simulink model "pendulum_control"  (R2025b)
settings: Solver=VariableStepAuto  StartTime=0.0  StopTime=4  RelTol=1e-3
undefined symbols (not defined in the file): b, K, Kd, Kp, Kt, L, R, setpoint
settings Model: Creator=REARDONNM24  LastModifiedBy=REARDONNM24

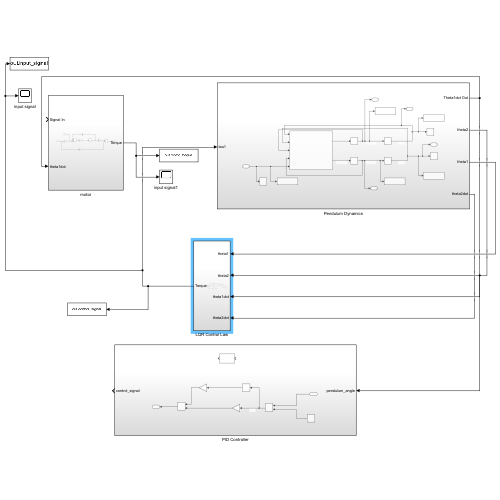
[thumbnail: Simulink's stored preview of the top-level diagram]
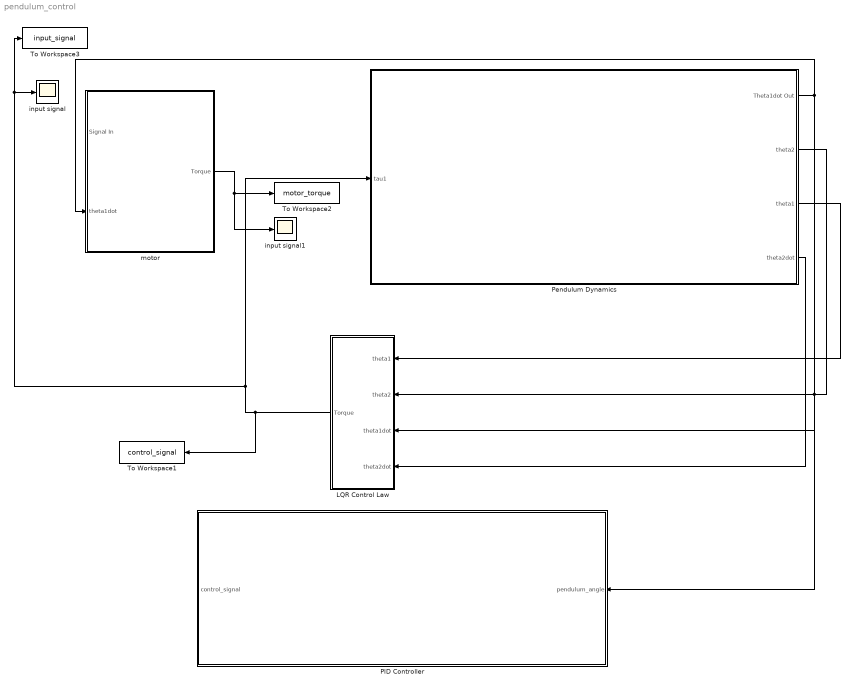
== system pendulum_control ==
  LQR Control Law : Subsystem
  PID Controller : Subsystem
      settings: PortSchema="{\"entries\":[{\"content\":{\"sides\":[{\"content\":{\"connectorIds\":[\"Out1\"]},\"type\":\"ConnectorPlacement.EquallySpacedRectSide\",\"uuid\":\"140972ef-afa4-4424-8e07-e9b39865205a\"},{\"content\":{\"connectorIds\":[\"In1\"],\"side\":\"RIGHT\"},\"type\":\"ConnectorPlacement.EquallySpacedRectSide\",\"uuid\":\"e18a6186-4364-4339-999d-66e09d6bd355\"},{\"content\":{\"side\":\"TOP\"},\"type\":\"ConnectorPlacement.EquallySpacedRectSide\",\"uuid\":\"cdbf3bcd-b810-497c-aa1d-b7994b8093ed\"}]},\"type\":\"ConnectorPlacement.EquallySpacedConnector\",\"uuid\":\"2c683edf-d322-406a-ba66-9fd9d67fa1ef\"}],\"packageUris\":[\"http://schema.mathworks.com/mf0/Connector/R2020b\"],\"version\":\"1.0\"}"
  Pendulum Dynamics : Subsystem
  To Workspace1 : ToWorkspace  VariableName=control_signal  SaveFormat=Timeseries  SampleTime=-1
  To Workspace2 : ToWorkspace  VariableName=motor_torque  SaveFormat=Timeseries  SampleTime=-1
  To Workspace3 : ToWorkspace  VariableName=input_signal  SaveFormat=Timeseries  SampleTime=-1
  input signal : Scope
      settings: ActiveDisplayYMinimum=174.41543511722466  ActiveDisplayYMaximum=4357.1108128089754  DataLoggingVariableName=ScopeData6
  input signal1 : Scope
      settings: ActiveDisplayYMinimum=-0.0033441907118329393  ActiveDisplayYMaximum=0.00610606731194419  DataLoggingVariableName=ScopeData7
  motor : Subsystem
  wires:
  Pendulum Dynamics/1(Theta1dot Out) -> motor/2(theta1dot), LQR Control Law/3(theta1dot)
  motor/1(Torque) -> input signal1/1, To Workspace2/1
  Pendulum Dynamics/2(theta2) -> LQR Control Law/2(theta2), PID Controller/1(pendulum_angle)
  Pendulum Dynamics/3(theta1) -> LQR Control Law/1(theta1)
  Pendulum Dynamics/4(theta2dot) -> LQR Control Law/4(theta2dot)
  LQR Control Law/1(Torque) -> To Workspace1/1, To Workspace3/1, input signal/1, Pendulum Dynamics/1(tau1)

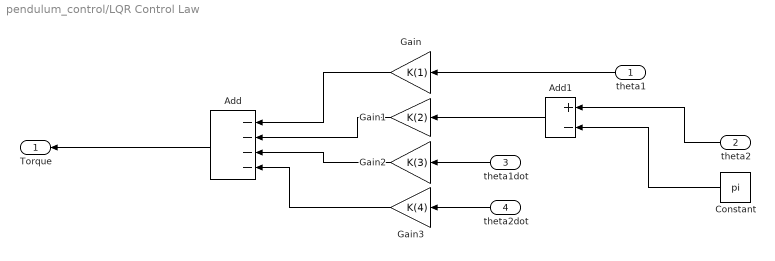
== system pendulum_control/LQR Control Law ==
  theta1 : Inport
  theta2 : Inport  Port=2
  theta1dot : Inport  Port=3
  theta2dot : Inport  Port=4
  Add : Sum  Inputs=----
  Add1 : Sum  Inputs=+-
  Constant : Constant  Value=pi
  Gain : Gain  Gain=K(1)
  Gain1 : Gain  Gain=K(2)
  Gain2 : Gain  Gain=K(3)
  Gain3 : Gain  Gain=K(4)
  Torque : Outport
  wires:
  Gain3/1 -> Add/4
  Gain/1 -> Add/1
  theta2dot/1 -> Gain3/1
  theta1dot/1 -> Gain2/1
  Gain1/1 -> Add/2
  Gain2/1 -> Add/3
  Add/1 -> Torque/1
  Constant/1 -> Add1/2
  theta2/1 -> Add1/1
  theta1/1 -> Gain/1
  Add1/1 -> Gain1/1

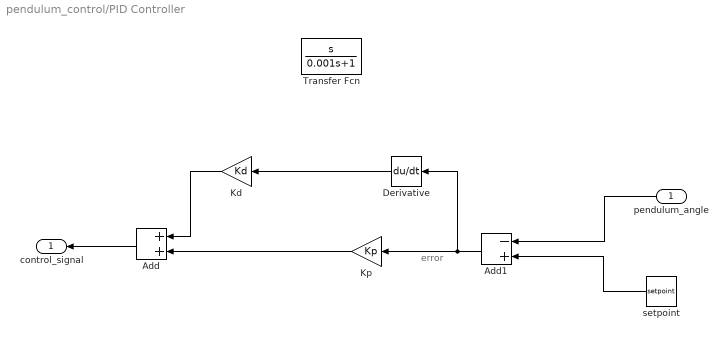
== system pendulum_control/PID Controller ==
  note: error
  pendulum_angle : Inport
  Add : Sum
  Add1 : Sum  Inputs=-+
  Derivative : Derivative
  Kd : Gain  Gain=Kd
  Kp : Gain  Gain=Kp
  Transfer Fcn : TransferFcn  Numerator=[1 0]  Denominator=[0.001 1]
  setpoint : Constant  Value=setpoint
  control_signal : Outport
  wires:
  Add1/1 -> Derivative/1, Kp/1
  setpoint/1 -> Add1/2
  pendulum_angle/1 -> Add1/1
  Kp/1 -> Add/2
  Kd/1 -> Add/1
  Add/1 -> control_signal/1
  Derivative/1 -> Kd/1

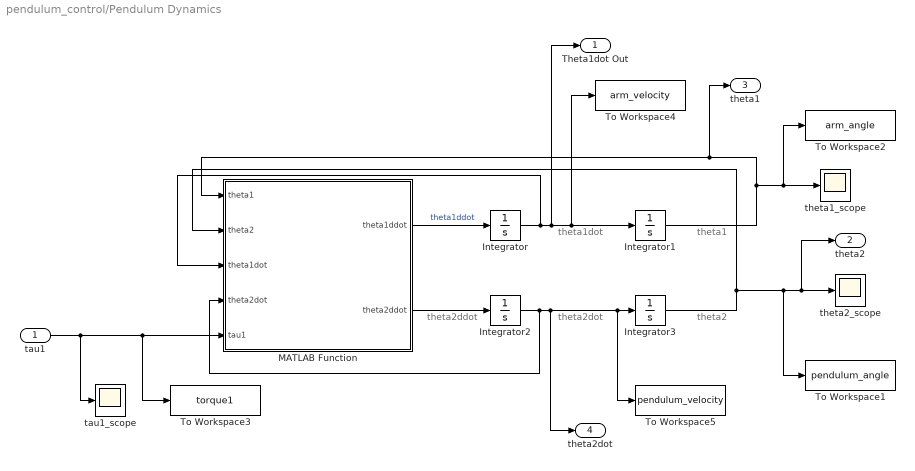
== system pendulum_control/Pendulum Dynamics ==
  note: theta1
  note: theta2
  note: theta2dot
  note: theta2ddot
  note: theta1dot
  tau1 : Inport
  Integrator : Integrator
  Integrator1 : Integrator
  Integrator2 : Integrator
  Integrator3 : Integrator  InitialCondition=2.96
  MATLAB Function : MATLAB Function  TreatAsAtomicUnit=on
  To Workspace1 : ToWorkspace  VariableName=pendulum_angle  SaveFormat=Timeseries  SampleTime=-1
  To Workspace2 : ToWorkspace  VariableName=arm_angle  SaveFormat=Timeseries  SampleTime=-1
  To Workspace3 : ToWorkspace  VariableName=torque1  SaveFormat=Timeseries  SampleTime=-1
  To Workspace4 : ToWorkspace  VariableName=arm_velocity  SaveFormat=Timeseries  SampleTime=-1
  To Workspace5 : ToWorkspace  VariableName=pendulum_velocity  SaveFormat=Timeseries  SampleTime=-1
  tau1_scope : Scope
      settings: ActiveDisplayYMinimum=-0.018770395001535239  ActiveDisplayYMaximum=0.012159767110327464  DataLoggingVariableName=ScopeData4
  theta1_scope : Scope
      settings: ActiveDisplayYMinimum=-0.0042282998397400089  ActiveDisplayYMaximum=0.03805469855766009  DataLoggingVariableName=ScopeData2
  theta2_scope : Scope
      settings: ActiveDisplayYMinimum=-1.85410777692418  ActiveDisplayYMaximum=-0.63109346273532874  DataLoggingVariableName=ScopeData3
  Theta1dot Out : Outport
  theta2 : Outport  Port=2
  theta1 : Outport  Port=3
  theta2dot : Outport  Port=4
  wires:
  MATLAB Function/1(theta1ddot) -> Integrator/1  "theta1ddot"
  Integrator/1 -> MATLAB Function/3(theta1dot), Theta1dot Out/1, Integrator1/1, To Workspace4/1
  Integrator2/1 -> MATLAB Function/4(theta2dot), theta2dot/1, To Workspace5/1, Integrator3/1
  MATLAB Function/2(theta2ddot) -> Integrator2/1
  Integrator3/1 -> To Workspace1/1, theta2/1, theta2_scope/1, MATLAB Function/2(theta2)
  Integrator1/1 -> To Workspace2/1, theta1_scope/1, theta1/1, MATLAB Function/1(theta1)
  tau1/1 -> tau1_scope/1, To Workspace3/1, MATLAB Function/5(tau1)

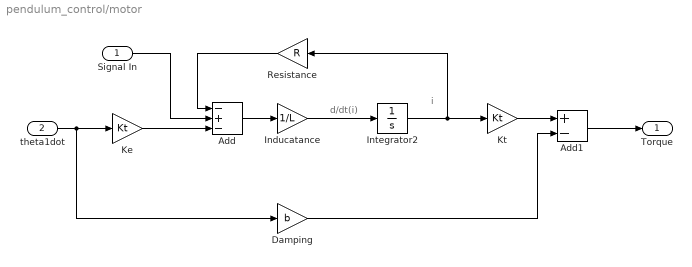
== system pendulum_control/motor ==
  note: i
  note: d/dt(i)
  Signal In : Inport
  theta1dot : Inport  Port=2
  Add : Sum  Inputs=-+-
  Add1 : Sum  Inputs=+-
  Damping : Gain  Gain=b
  Inducatance : Gain  Gain=1/L
  Integrator2 : Integrator
  Ke : Gain  Gain=Kt
  Kt : Gain  Gain=Kt
  Resistance : Gain  Gain=R
  Torque : Outport
  wires:
  Signal In/1 -> Add/2
  Resistance/1 -> Add/1
  Integrator2/1 -> Kt/1, Resistance/1
  Inducatance/1 -> Integrator2/1
  Add/1 -> Inducatance/1
  Ke/1 -> Add/3
  theta1dot/1 -> Damping/1, Ke/1
  Kt/1 -> Add1/1
  Damping/1 -> Add1/2
  Add1/1 -> Torque/1

== matlab function pendulum_control/Pendulum Dynamics/MATLAB Function ==
  data: theta1 input; theta1ddot output; theta2 input; theta1dot input; theta2dot input; tau1 input; theta2ddot output
function [theta1ddot, theta2ddot] = pendulum_dynamics(theta1, theta2, theta1dot, theta2dot, tau1)
    % Define constants
    L1 = 0.03;
    L2 = 0.07;
    l1 = L1/2;
    l2 = L2/2;
    m1 = 1e-3;
    m2 = 5e-3;
    J1 = 1/3 * m1 * L1^2;
    J2 = 1/3 * m2 * L2^2;
    b1 = 1e-5;
    b2 = 1e-5;
    g = 9.81;

    % assume the following for now:
    J1xx = 0;
    J1yy = J1;
    J1zz = J1;
    J2xx = 0;
    J2yy = J2;
    J2zz = J2;

    % define the mass matrix
    M11 = J1zz + m1*l1^2 + m2*L1^2 + (J2yy+m2*l2^2)*sin(theta2)^2 + J2xx*cos(theta2)^2;
    M12 = m2*L1*l2*cos(theta2);
    M22 = m2*l2^2 + J2zz;

    M = [M11, M12; M12, M22];
    
    h1 = -m2*L1*l2*sin(theta2)*theta2dot^2 + theta1dot*theta2dot*sin(2*theta2)*(m2*l2^2 + J2yy - J2xx) + b1*theta1dot;
    h2 = 0.5*theta1dot^2*sin(2*theta2)*(-m2*l2^2 - J2yy + J2xx) + b2*theta2dot + g*m2*l2*sin(theta2);
    

    tau = [tau1; 0];

        
    qdd = M\(tau - [h1;h2]);

    theta1ddot = qdd(1);
    theta2ddot = qdd(2);
  

end
